simulink model "sampleModel1749"  (R2023a)
settings: Solver=VariableStepAuto  StartTime=0.0  StopTime=10.0  RelTol=1e-3
libraries: hdlsllib x3, simulink x3
settings Model: Creator=user1  LastModifiedBy=user1

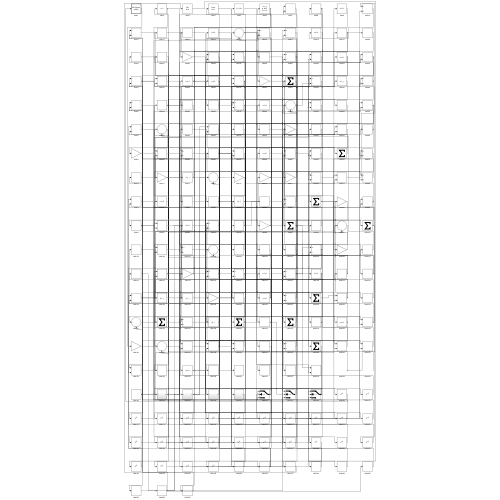
[thumbnail: Simulink's stored preview of the top-level diagram]
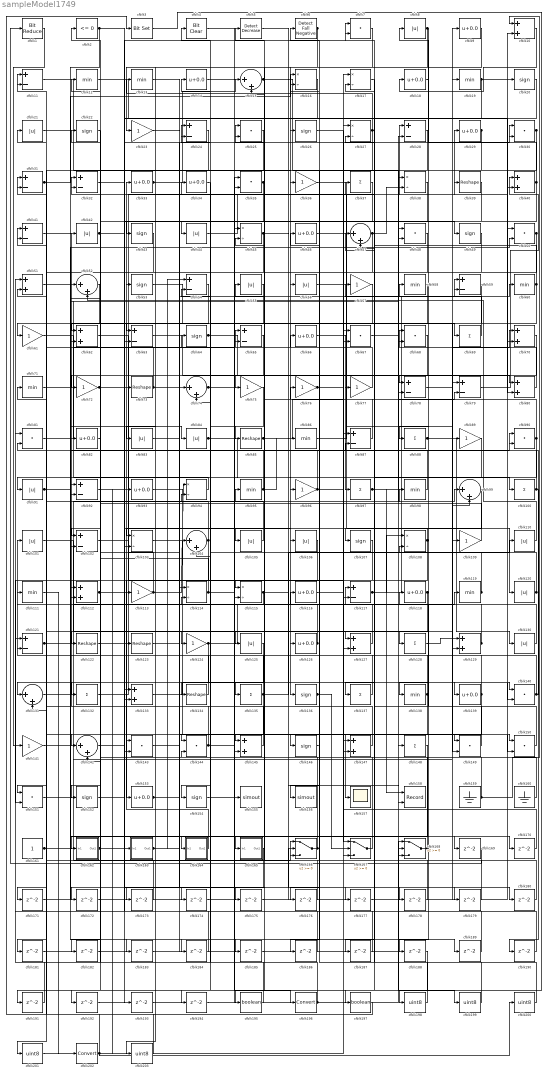
== system sampleModel1749 ==
  cfblk1 : hdlsllib/Logic and Bit Operations/Bit Reduce  mode=AND
  cfblk{10,40,51,62,70,80,112,127,129,133,145,147} (12 alike) : Sum
  cfblk{37,69,88,97,100,128,132,135,137,148} (10 alike) : Sum  Inputs=+
  cfblk{8,21,42,44,55..56,83..84,91,101,105..106,110,120,125,130} (16 alike) : Abs  SaturateOnIntegerOverflow=off
  cfblk{11,24,28,31..32,41,54,59,63,65,78..79,87,92,102,117,121} (17 alike) : Sum  Inputs=+-
  cfblk{16..17,27,38,45,94,103,108,114..115} (10 alike) : Product  Inputs=*/  RndMeth=Zero  SaturateOnIntegerOverflow=on
  cfblk{15,47,52,74,99,104,131,142} (8 alike) : Sum  Inputs=|++
  cfblk{20,22,26,43,49,53,64,107,136,146,152,154} (12 alike) : Signum
  cfblk{23,36,57,61,72,75..77,89,96,109,113,124,141} (14 alike) : Gain
  cfblk{12..13,19,58,60,71,86,95,98,111,119,138} (12 alike) : MinMax
  cfblk{9,14,18,29,33..34,46,66,82,93,116,118,126,139,153} (15 alike) : Bias  Bias=0.0  SaturateOnIntegerOverflow=off
  cfblk{39,73,85,122..123,134} (6 alike) : Reshape
  cfblk{7,25,30,35,48,50,67..68,81,90,140,143..144,149..151} (16 alike) : DotProduct  OutDataTypeStr=Inherit: Inherit via internal rule
  cfblk155 : ToWorkspace  VariableName=simout  SaveFormat=Timeseries  SampleTime=-1
  cfblk156 : ToWorkspace  VariableName=simout  SaveFormat=Timeseries  SampleTime=-1
  cfblk157 : Scope
  cfblk158 : Record  FileSettingsInternal="{\"entries\":[{\"content\":{\"excelSettings\":{\"content\":{},\"type\":\"Streamout.ExcelSettings\"}},\"type\":\"Streamout.FileSettingStorage\",\"uuid\":\"\"}],\"packageUris\":[\"http:\\/\\/schema.mathworks.com\\/mf0\\/streamout_blocks\\/R2020a\"],\"version\":\"1.0\"}"  Layout=[1 1]  SignalsInternal="{\"entries\":[{\"content\":{},\"type\":\"RecordBlkView.InputSignals\",\"uuid\":\"\"}],\"packageUris\":[\"http:\\/\\/schema.mathworks.com\\/mf0\\/streamout_blocks\\/R2020a\"],\"version\":\"1.0\"}"  VisualizationBindings="{\"xyplotplugin\":{\"info\":[{\"series\":[{\"bindingParametersList\":[{\"parameter\":\"X-Axis\",\"signalID\":3706,\"signalName\":\"cfblk97\"},{\"parameter\":\"Y-Axis\",\"signalID\":3710,\"signalName\":\"cfblk85\"}],\"seriesID\":10306}],\"subplotID\":1}]}}"  CompatibilityTag=XY  st=-1
  cfblk159 : Ground
  cfblk160 : Ground
  cfblk161 : Constant  SampleTime=-1
  cfblk162 : Subsystem
      settings: LibrarySourceBlock=|
      | hdlsllib/Ports &
      | Subsystems/Subsystem
  cfblk163 : Subsystem
      settings: LibrarySourceBlock=|
      | hdlsllib/Ports &
      | Subsystems/Subsystem
  cfblk164 : Subsystem
      settings: LibrarySourceBlock=|
      | hdlsllib/Ports &
      | Subsystems/Subsystem
  cfblk165 : Subsystem
      settings: LibrarySourceBlock=|
      | hdlsllib/Ports &
      | Subsystems/Subsystem
  cfblk166 : Switch  SaturateOnIntegerOverflow=off  InputSameDT=off
  cfblk167 : Switch  SaturateOnIntegerOverflow=off  InputSameDT=off
  cfblk168 : Switch  SaturateOnIntegerOverflow=off  InputSameDT=off
  cfblk{169..194} (26 alike) : Delay  SampleTime=1
  cfblk195 : DataTypeConversion  OutDataTypeStr=boolean  SaturateOnIntegerOverflow=off  RndMeth=Floor
  cfblk196 : DataTypeConversion  SaturateOnIntegerOverflow=off  RndMeth=Floor
  cfblk197 : DataTypeConversion  OutDataTypeStr=boolean  SaturateOnIntegerOverflow=off  RndMeth=Floor
  cfblk{198..201,203} (5 alike) : DataTypeConversion  OutDataTypeStr=uint8  SaturateOnIntegerOverflow=off  RndMeth=Floor
  cfblk2 : hdlsllib/Logic and Bit Operations/Compare To Zero  relop=<=  OutDataTypeStr=boolean
  cfblk202 : DataTypeConversion  SaturateOnIntegerOverflow=off  RndMeth=Floor
  cfblk3 : simulink/Logic and Bit Operations/Bit Set  iBit=0
      settings: LibrarySourceBlock=|
      | hdlsllib/Logic and Bit
      | Operations/Bit Set
  cfblk4 : simulink/Logic and Bit Operations/Bit Clear  iBit=0
      settings: LibrarySourceBlock=|
      | hdlsllib/Logic and Bit
      | Operations/Bit Clear
  cfblk5 : simulink/Logic and Bit Operations/Detect Decrease  vinit=0.0  OutDataTypeStr=boolean
      settings: LibrarySourceBlock=|
      | hdlsllib/Logic and Bit
      | Operations/Detect
      | Decrease
  cfblk6 : hdlsllib/Logic and Bit Operations/Detect Fall Negative  vinit=0  OutDataTypeStr=boolean
  wires:
  cfblk163/1(Out1) -> cfblk74/1, cfblk59/2, cfblk54/1
  cfblk140/1 -> cfblk32/1, cfblk90/2
  cfblk88/1 -> cfblk130/1, cfblk99/2
  cfblk134/1 -> cfblk101/1
  cfblk101/1 -> cfblk128/1
  cfblk9/1 -> cfblk136/1
  cfblk161/1 -> cfblk166/1, cfblk9/1
  cfblk34/1 -> cfblk144/1
  cfblk131/1 -> cfblk119/1
  cfblk112/1 -> cfblk30/2, cfblk174/1
  cfblk10/1 -> cfblk18/1
  cfblk117/1 -> cfblk59/1, cfblk108/1
  cfblk121/1 -> cfblk95/1, cfblk53/1
  cfblk144/1 -> cfblk42/1, cfblk90/1
  cfblk127/1 -> cfblk117/1
  cfblk41/1 -> cfblk69/1
  cfblk84/1 -> cfblk96/1, cfblk38/1, cfblk54/2
  cfblk139/1 -> cfblk71/1, cfblk142/2
  cfblk79/1 -> cfblk40/1
  cfblk159/1 -> cfblk10/1, cfblk81/2
  cfblk104/1 -> cfblk31/1, cfblk151/2
  cfblk1/1 -> cfblk141/1
  cfblk63/1 -> cfblk75/1
  cfblk153/1 -> cfblk178/1, cfblk179/1
  cfblk167/1 -> cfblk66/1
  cfblk48/1 -> cfblk115/1
  cfblk164/1(Out1) -> cfblk33/1
  cfblk36/1 -> cfblk80/1
  cfblk150/1 -> cfblk37/1
  cfblk132/1 -> cfblk98/1
  cfblk40/1 -> cfblk8/1, cfblk147/2
  cfblk151/1 -> cfblk48/1
  cfblk109/1 -> cfblk2/1
  cfblk99/1 -> cfblk107/1
  cfblk18/1 -> cfblk88/1
  cfblk49/1 -> cfblk146/1
  cfblk39/1 -> cfblk105/1
  cfblk21/1 -> cfblk36/1
  cfblk61/1 -> cfblk148/1
  cfblk102/1 -> cfblk29/1
  cfblk44/1 -> cfblk28/1
  cfblk137/1 -> cfblk52/1
  cfblk122/1 -> cfblk10/2
  cfblk110/1 -> cfblk52/2
  cfblk31/1 -> cfblk16/1, cfblk170/1
  cfblk120/1 -> cfblk74/2, cfblk17/2
  cfblk133/1 -> cfblk139/1
  cfblk116/1 -> cfblk60/1
  cfblk113/1 -> cfblk94/1, cfblk62/2
  cfblk35/1 -> cfblk102/1, cfblk44/1
  cfblk81/1 -> cfblk28/2
  cfblk103/1 -> cfblk157/1
  cfblk37/1 -> cfblk85/1
  cfblk60/1 -> cfblk134/1, cfblk32/2
  cfblk136/1 -> cfblk46/1, cfblk167/2
  cfblk130/1 -> cfblk5/1
  cfblk4/1 -> cfblk196/1
  cfblk62/1 -> cfblk117/2
  cfblk107/1 -> cfblk153/1
  cfblk128/1 -> cfblk129/1
  cfblk108/1 -> cfblk103/1, cfblk122/1, cfblk176/1
  cfblk2/1 -> cfblk92/2, cfblk26/1
  cfblk6/1 -> cfblk23/1, cfblk203/1
  cfblk46/1 -> cfblk120/1
  cfblk118/1 -> cfblk137/1, cfblk171/1
  cfblk33/1 -> cfblk15/1, cfblk127/2
  cfblk11/1 -> cfblk104/1
  cfblk73/1 -> cfblk168/2, cfblk41/1
  cfblk119/1 -> cfblk55/1, cfblk57/1
  cfblk45/1 -> cfblk129/2, cfblk152/1
  cfblk168/1 -> cfblk27/2, cfblk162/1(In1)
  cfblk90/1 -> cfblk138/1, cfblk65/2
  cfblk106/1 -> cfblk126/1
  cfblk47/1 -> cfblk154/1, cfblk38/2
  cfblk51/1 -> cfblk84/1
  cfblk105/1 -> cfblk64/1
  cfblk70/1 -> cfblk132/1
  cfblk147/1 -> cfblk82/1
  cfblk143/1 -> cfblk150/1
  cfblk66/1 -> cfblk97/1
  cfblk93/1 -> cfblk155/1
  cfblk124/1 -> cfblk89/1, cfblk151/1, cfblk99/1
  cfblk38/1 -> cfblk125/1
  cfblk96/1 -> cfblk100/1, cfblk41/2
  cfblk78/1 -> cfblk70/1
  cfblk65/1 -> cfblk123/1
  cfblk166/1 -> cfblk14/1, cfblk116/1
  cfblk97/1 -> cfblk79/2, cfblk158/1
  cfblk125/1 -> cfblk143/1
  cfblk135/1 -> cfblk110/1, cfblk112/2, cfblk181/1
  cfblk114/1 -> cfblk58/1, cfblk22/1
  cfblk55/1 -> cfblk124/1
  cfblk52/1 -> cfblk61/1
  cfblk74/1 -> cfblk164/1(In1), cfblk140/2
  cfblk76/1 -> cfblk6/1, cfblk150/2
  cfblk29/1 -> cfblk133/2, cfblk68/2
  cfblk91/1 -> cfblk50/2, cfblk183/1
  cfblk25/1 -> cfblk83/1
  cfblk32/1 -> cfblk73/1
  cfblk83/1 -> cfblk149/1
  cfblk26/1 -> cfblk147/1
  cfblk86/1 -> cfblk19/1
  cfblk16/1 -> cfblk35/2
  cfblk154/1 -> cfblk39/1
  cfblk12/1 -> cfblk70/2
  cfblk148/1 -> cfblk165/1(In1)
  cfblk145/1 -> cfblk121/2
  cfblk7/1 -> cfblk43/1
  cfblk98/1 -> cfblk65/1
  cfblk58/1 -> cfblk135/1
  cfblk87/1 -> cfblk76/1
  cfblk82/1 -> cfblk142/1
  cfblk138/1 -> cfblk143/2, cfblk25/2
  cfblk94/1 -> cfblk91/1
  cfblk56/1 -> cfblk109/1
  cfblk30/1 -> cfblk62/1, cfblk80/2
  cfblk111/1 -> cfblk202/1
  cfblk80/1 -> cfblk68/1
  cfblk13/1 -> cfblk145/1
  cfblk27/1 -> cfblk13/1, cfblk127/1, cfblk72/1
  cfblk100/1 -> cfblk24/1, cfblk190/1
  cfblk92/1 -> cfblk94/2
  cfblk57/1 -> cfblk156/1
  cfblk69/1 -> cfblk7/1
  cfblk20/1 -> cfblk63/1
  cfblk14/1 -> cfblk140/1
  cfblk71/1 -> cfblk45/1
  cfblk160/1 -> cfblk15/2
  cfblk72/1 -> cfblk106/1, cfblk7/2
  cfblk19/1 -> cfblk103/2, cfblk20/1, cfblk47/2
  cfblk8/1 -> cfblk188/1, cfblk195/1
  cfblk85/1 -> cfblk17/1, cfblk158/2
  cfblk95/1 -> cfblk11/1, cfblk86/1
  cfblk24/1 -> cfblk131/1
  cfblk162/1(Out1) -> cfblk63/2, cfblk30/1
  cfblk141/1 -> cfblk87/2
  cfblk149/1 -> cfblk118/1
  cfblk77/1 -> cfblk21/1
  cfblk129/1 -> cfblk25/1, cfblk51/2
  cfblk53/1 -> cfblk149/2
  cfblk42/1 -> cfblk49/1, cfblk185/1
  cfblk115/1 -> cfblk114/2, cfblk108/2
  cfblk28/1 -> cfblk56/1
  cfblk50/1 -> cfblk115/2, cfblk173/1
  cfblk68/1 -> cfblk78/1
  cfblk126/1 -> cfblk34/1, cfblk113/1
  cfblk64/1 -> cfblk167/1, cfblk77/1, cfblk189/1
  cfblk15/1 -> cfblk48/2, cfblk78/2
  cfblk23/1 -> cfblk169/1
  cfblk169/1 -> cfblk1/1
  cfblk170/1 -> cfblk27/1
  cfblk171/1 -> cfblk102/2
  cfblk165/1(Out1) -> cfblk172/1
  cfblk172/1 -> cfblk166/2
  cfblk173/1 -> cfblk11/2
  cfblk174/1 -> cfblk50/1
  cfblk59/1 -> cfblk175/1
  cfblk175/1 -> cfblk40/2
  cfblk176/1 -> cfblk31/2
  cfblk5/1 -> cfblk177/1
  cfblk177/1 -> cfblk79/1
  cfblk178/1 -> cfblk92/1
  cfblk179/1 -> cfblk45/2
  cfblk123/1 -> cfblk180/1
  cfblk180/1 -> cfblk112/1
  cfblk181/1 -> cfblk167/3
  cfblk22/1 -> cfblk182/1
  cfblk182/1 -> cfblk114/1
  cfblk183/1 -> cfblk145/2
  cfblk142/1 -> cfblk184/1
  cfblk184/1 -> cfblk121/1
  cfblk185/1 -> cfblk168/3
  cfblk146/1 -> cfblk186/1
  cfblk186/1 -> cfblk24/2
  cfblk17/1 -> cfblk187/1
  cfblk187/1 -> cfblk133/1
  cfblk189/1 -> cfblk16/2
  cfblk190/1 -> cfblk104/2
  cfblk43/1 -> cfblk191/1
  cfblk191/1 -> cfblk51/1
  cfblk54/1 -> cfblk192/1
  cfblk192/1 -> cfblk35/1
  cfblk152/1 -> cfblk193/1
  cfblk193/1 -> cfblk87/1
  cfblk75/1 -> cfblk194/1
  cfblk194/1 -> cfblk168/1
  cfblk195/1 -> cfblk4/1
  cfblk196/1 -> cfblk144/2, cfblk12/1, cfblk81/1
  cfblk89/1 -> cfblk197/1
  cfblk197/1 -> cfblk3/1
  cfblk3/1 -> cfblk198/1
  cfblk198/1 -> cfblk47/1
  cfblk67/1 -> cfblk199/1
  cfblk199/1 -> cfblk166/3
  cfblk200/1 -> cfblk67/1
  cfblk188/1 -> cfblk201/1
  cfblk201/1 -> cfblk67/2
  cfblk202/1 -> cfblk200/1, cfblk93/1, cfblk131/2, cfblk163/1(In1)
  cfblk203/1 -> cfblk111/1

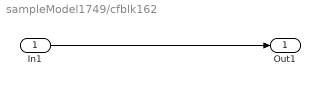
== system sampleModel1749/cfblk162 ==
  In1 : Inport
  Out1 : Outport
  wires:
  In1/1 -> Out1/1

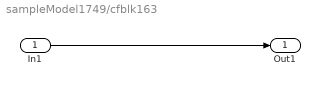
== system sampleModel1749/cfblk163 ==
  In1 : Inport
  Out1 : Outport
  wires:
  In1/1 -> Out1/1

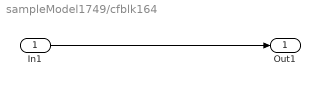
== system sampleModel1749/cfblk164 ==
  In1 : Inport
  Out1 : Outport
  wires:
  In1/1 -> Out1/1

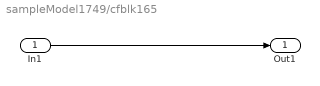
== system sampleModel1749/cfblk165 ==
  In1 : Inport
  Out1 : Outport
  wires:
  In1/1 -> Out1/1
